simulink model "data_acquisition"  (R2026a)
settings: Solver=FixedStepAuto  StopTime=10  FixedStep=0.01  EnableMultiTasking=on
libraries: arduinolib x2, arduinosensorlib x1
settings Model: FPTRunName=Active  SILPILModeSetting=veronly  ExtModeTrigDuration=2  Creator=Nitro 5  LastModifiedBy=Adham
settings OptimizationCC: LifeSpan=Inf
settings DebuggingCC: UnderspecifiedInitializationDetection=Classic
settings HardwareCC: ProdLargestAtomicInteger=Long  ProdLargestAtomicFloat=Double  ProdHWDeviceType=ARM Compatible->ARM Cortex  UseEmbeddedCoderFeatures=off
settings RTWCC: SystemTargetFile=ert.tlc  HardwareBoard=ESP32-WROOM (Arduino Compatible)  GenerateReport=on  RTWVerbose=off  Toolchain=ESP32  BuildConfiguration=Faster Runs  LaunchReport=on  Description=Embedded Coder
settings CodeAppCC: MATLABSourceComments=on
settings ERTTargetCC: ExtModeTransport=3.0  ExtModeAutomaticAllocSize=off  ExtModeStaticAllocSize=65536.0  DynamicArrayContainerType=coder::array  MultiwordLength=2048.0  ERTCustomFileBanners=off  SupportContinuousTime=on  SupportNonInlinedSFcns=on  SupportVariableSizeSignals=on  ModelStepFunctionPrototypeControlCompliant=off
settings SimscapeCC: SimscapeNominalValues="[{\"value\":\"1\",\"unit\":\"A\"},{\"value\":\"1\",\"unit\":\"bar\"},{\"value\":\"1\",\"unit\":\"cm^2\"},{\"value\":\"1\",\"unit\":\"cm^3/s\"},{\"value\":\"1\",\"unit\":\"kJ/kg\"},{\"value\":\"1\",\"unit\":\"kW\"},{\"value\":\"1\",\"unit\":\"l\"},{\"value\":\"1\",\"unit\":\"N\"},{\"value\":\"1\",\"unit\":\"N*m\"},{\"value\":\"1\",\"unit\":\"V\"}]"  SimscapeLogType=none  SimscapeLogDataHistory=5000.0

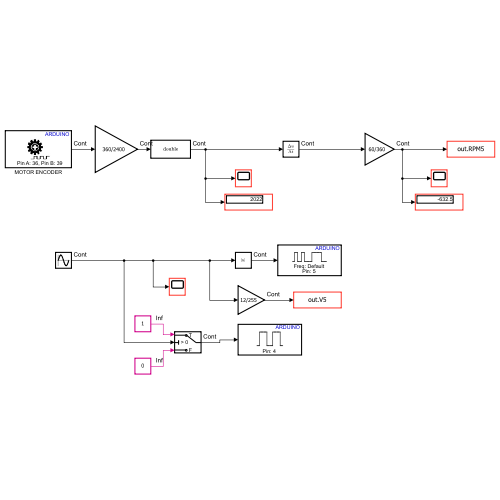
[thumbnail: Simulink's stored preview of the top-level diagram]
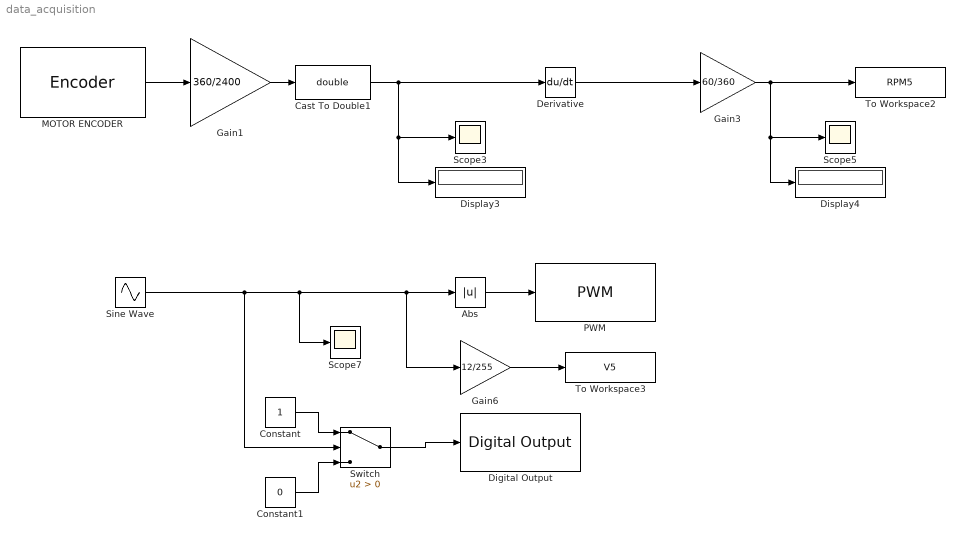
== system data_acquisition ==
  Abs : Abs  SaturateOnIntegerOverflow=off
  Cast To Double1 : DataTypeConversion  OutDataTypeStr=double  SaturateOnIntegerOverflow=off  RndMeth=Floor
  Constant : Constant
  Constant1 : Constant  Value=0
  Derivative : Derivative
  Digital Output : arduinolib/Digital Output  pinNumber=4  Direction=output  blockPlatform=arduino
  Display3 : Display
  Display4 : Display
  Gain1 : Gain  Gain=360/2400
  Gain3 : Gain  Gain=60/360
  Gain6 : Gain  Gain=12/255
  MOTOR ENCODER : arduinosensorlib/Encoder  InputA=36  InputB=39  Mode=No reset  SampleTime=-1
  PWM : arduinolib/PWM  pinNumber=5  frequencyType=Default  desiredFrequency=490.2  achievableFrequency=490.2
  Scope3 : Scope
      settings: ActiveDisplayYMinimum=-725.38125011259388  ActiveDisplayYMaximum=6528.4312510133459  DataLoggingVariableName=ScopeData3
  Scope5 : Scope
      settings: ActiveDisplayYMinimum=-2135.0000003312512  ActiveDisplayYMaximum=2240.0000003475425  DataLoggingVariableName=ScopeData5
  Scope7 : Scope
      settings: ActiveDisplayYMinimum=-62.49889824414749  ActiveDisplayYMaximum=62.494980921975682  DataLoggingVariableName=ScopeData7
  Sine Wave : Sin  Amplitude=150  Frequency=5  SampleTime=0
  Switch : Switch  Criteria=u2 > Threshold  SaturateOnIntegerOverflow=off  InputSameDT=off
  To Workspace2 : ToWorkspace  VariableName=RPM5  SampleTime=-1
      settings: Save2DSignal=2-D array (concatenate along first dimension)
  To Workspace3 : ToWorkspace  VariableName=V5  SampleTime=-1
      settings: Save2DSignal=2-D array (concatenate along first dimension)
  wires:
  MOTOR ENCODER/1 -> Gain1/1
  Switch/1 -> Digital Output/1
  Constant/1 -> Switch/1
  Constant1/1 -> Switch/3
  Gain3/1 -> To Workspace2/1, Scope5/1, Display4/1
  Gain1/1 -> Cast To Double1/1
  Derivative/1 -> Gain3/1
  Cast To Double1/1 -> Derivative/1, Display3/1, Scope3/1
  Gain6/1 -> To Workspace3/1
  Abs/1 -> PWM/1
  Sine Wave/1 -> Abs/1, Gain6/1, Scope7/1, Switch/2
